simulink model "ModelEquationsDOF2"  (R2022b)
settings: Solver=ode4  StartTime=0.0  StopTime=100  FixedStep=10^-3  RelTol=1e-3
values from neighbouring files (symbols this model uses):
  cs = 900    [OptimizedParamDOF2.m]
  cu = 850    [ModelFixedParamDOF2.m]
  ks = 10039    [OptimizedParamDOF2.m]
  ku = 150000    [ModelFixedParamDOF2.m]
  ms = 237    [ModelFixedParamDOF2.m]    (also in ModelFixedParamDOF3.m = 35; ModelFixedParamDOF5.m = 730)
  mu = 20    [ModelFixedParamDOF2.m]
  road_front_wheel = M.'    [LoadRoadScript.m]
settings Model: Creator=Ade  LastModifiedBy=andre
settings SolverCC: AlgebraicLoopSolver=TrustRegion
settings DataIOCC: ReturnWorkspaceOutputs=off
settings DebuggingCC: UnconnectedInputMsg=warning  UnconnectedOutputMsg=warning  UnconnectedLineMsg=warning  SFMachineParentedDataDiag=warning  ArithmeticOperatorsInVariantConditions=warning
settings ModelReferenceCC: EnableRefExpFcnMdlSchedulingChecks=on
settings SFSimCC: SimUseLocalCustomCode=off  CustomCodeUndefinedFunction=UseInterfaceOnly
settings RTWCC: RTWUseLocalCustomCode=off  DLArmComputeVersion=19.05

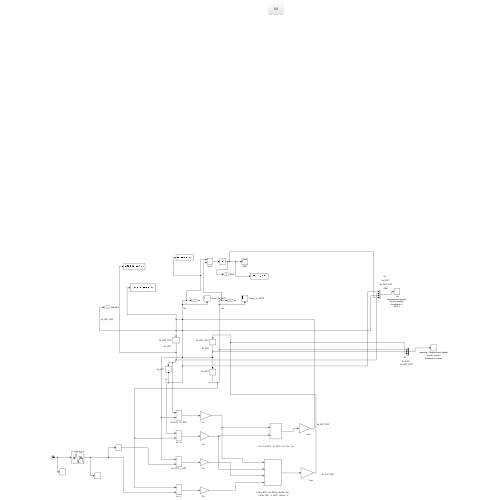
[thumbnail: Simulink's stored preview of the top-level diagram]
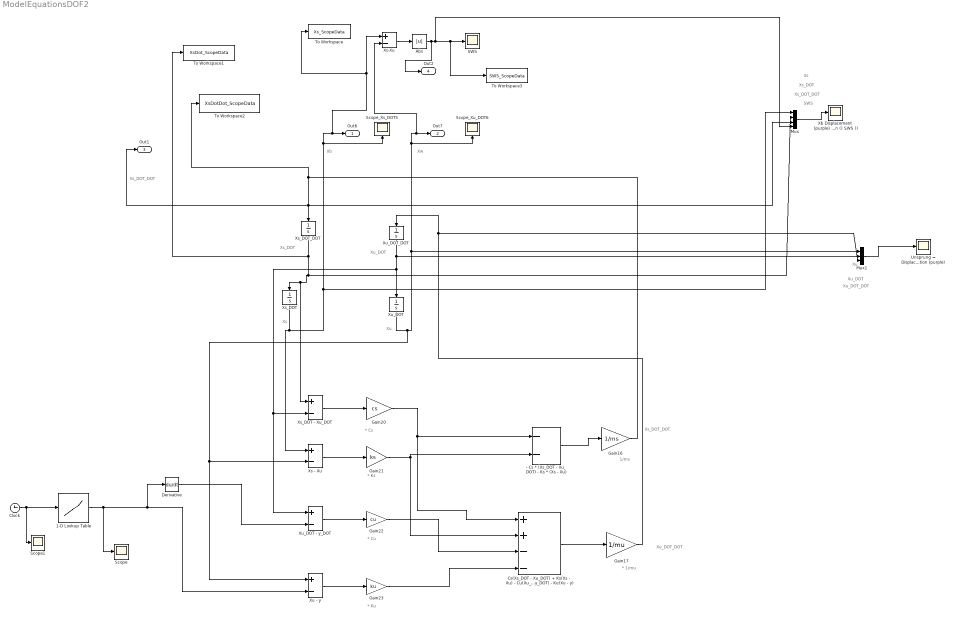
== system ModelEquationsDOF2 ==
  note: Xu_DOT_DOT
  note: * 1/mu
  note: Xs
  note: Xs_DOT
  note: Xu
  note: Xu_DOT
  note: Xu_DOT_DOT
  note: Xs_DOT_DOT
  note: 1/ms
  note: Xb
  note: Xw
  note: Xs_DOT_DOT
  note: * Ku
  note: * Cu
  note: * Cs
  note: * Ks
  note: Xu_DOT
  note: Xu
  note: Xs
  note: Xs_DOT
  note: Xs_DOT_DOT
  note: SWS
  " Cs(Xs_DOT - Xu_DOT) + Ks(Xs - Xu) - Cu(Xu_DOT - y_DOT) - Ku(Xu - y)" : Sum  Inputs=++--
  " - Cs * (Xs_DOT - Xu_DOT) - Ks * (Xs - Xu)" : Sum  Inputs=--
  "  Xb Displacement (purple) Velocity (purple) Acceleration () SWS ()" : Scope
  1-D Lookup Table : Lookup_n-D  NumberOfTableDimensions=1  LookupTableObject=road_front_wheel  BreakpointsForDimension1=[1:100]  Table=road_front_wheel  InternalRulePriority=Speed  RndMeth=Simplest
  Abs : Abs  SaturateOnIntegerOverflow=off
  Clock : Clock
  Derivative : Derivative
  Gain16 : Gain  Gain=1/ms
  Gain17 : Gain  Gain=1/mu
  Gain20 : Gain  Gain=cs
  Gain21 : Gain  Gain=ks
  Gain22 : Gain  Gain=cu
  Gain23 : Gain  Gain=ku
  Mux : Mux
  Mux1 : Mux  Inputs=3
  SWS : Scope
  Scope : Scope
  Scope1 : Scope
  Scope_Xs_DOT5 : Scope
  Scope_Xu_DOT6 : Scope
  To Workspace : ToWorkspace  VariableName=Xs_ScopeData  SaveFormat=Structure With Time  SampleTime=-1
  To Workspace1 : ToWorkspace  VariableName=XsDot_ScopeData  SaveFormat=Structure With Time  SampleTime=-1
  To Workspace2 : ToWorkspace  VariableName=XsDotDot_ScopeData  SaveFormat=Structure With Time  SampleTime=-1
  To Workspace3 : ToWorkspace  VariableName=SWS_ScopeData  SaveFormat=Structure With Time  SampleTime=-1
  Unsprung = Displacement (yellow) Velocity (purple) Acceleration (purple) : Scope
  Xs - Xu : Sum  Inputs=+-
  Xs-Xu : Sum  Inputs=+-
  Xs_DOT : Integrator
  Xs_DOT - Xu_DOT : Sum  Inputs=+-
  Xs_DOT_DOT : Integrator
  Xu - y : Sum  Inputs=+-
  "Xu_DOT " : Integrator
  "Xu_DOT - y_DOT " : Sum  Inputs=+-
  "Xu_DOT_DOT " : Integrator
  Out6 : Outport  SignalName=Xs  VectorParamsAs1DForOutWhenUnconnected=off
  Out7 : Outport  Port=2  SignalName=Xu  VectorParamsAs1DForOutWhenUnconnected=off
  Out1 : Outport  Port=3  SignalName=XsDotDot  VectorParamsAs1DForOutWhenUnconnected=off
  Out2 : Outport  Port=4  SignalName=SWS  VectorParamsAs1DForOutWhenUnconnected=off
  wires:
  Xs_DOT/1 -> Mux/1, To Workspace/1, Xs-Xu/1, Out6/1, Scope_Xs_DOT5/1, Xs - Xu/1
  " - Cs * (Xs_DOT - Xu_DOT) - Ks * (Xs - Xu)"/1 -> Gain16/1
  " Cs(Xs_DOT - Xu_DOT) + Ks(Xs - Xu) - Cu(Xu_DOT - y_DOT) - Ku(Xu - y)"/1 -> Gain17/1
  Xs - Xu/1 -> Gain21/1
  Xs_DOT - Xu_DOT/1 -> Gain20/1
  Xu - y/1 -> Gain23/1
  "Xu_DOT - y_DOT "/1 -> Gain22/1
  Gain23/1 -> " Cs(Xs_DOT - Xu_DOT) + Ks(Xs - Xu) - Cu(Xu_DOT - y_DOT) - Ku(Xu - y)"/4
  Gain22/1 -> " Cs(Xs_DOT - Xu_DOT) + Ks(Xs - Xu) - Cu(Xu_DOT - y_DOT) - Ku(Xu - y)"/3
  Gain21/1 -> " - Cs * (Xs_DOT - Xu_DOT) - Ks * (Xs - Xu)"/2, " Cs(Xs_DOT - Xu_DOT) + Ks(Xs - Xu) - Cu(Xu_DOT - y_DOT) - Ku(Xu - y)"/2
  Gain20/1 -> " - Cs * (Xs_DOT - Xu_DOT) - Ks * (Xs - Xu)"/1, " Cs(Xs_DOT - Xu_DOT) + Ks(Xs - Xu) - Cu(Xu_DOT - y_DOT) - Ku(Xu - y)"/1
  "Xu_DOT_DOT "/1 -> "Xu_DOT "/1, "Xu_DOT - y_DOT "/1, Xs_DOT - Xu_DOT/2, Mux1/2
  Gain16/1 -> Out1/1, Xs_DOT_DOT/1, Mux/3, To Workspace2/1
  Gain17/1 -> "Xu_DOT_DOT "/1, Mux1/3
  1-D Lookup Table/1 -> Scope/1, Derivative/1, Xu - y/2
  "Xu_DOT "/1 -> Mux1/1, Xs-Xu/2, Out7/1, Scope_Xu_DOT6/1, Xu - y/1, Xs - Xu/2
  Xs-Xu/1 -> Abs/1
  Mux/1 -> "  Xb Displacement (purple) Velocity (purple) Acceleration () SWS ()"/1
  Mux1/1 -> Unsprung = Displacement (yellow) Velocity (purple) Acceleration (purple)/1
  Xs_DOT_DOT/1 -> Xs_DOT - Xu_DOT/1, Xs_DOT/1, Mux/2, To Workspace1/1
  Clock/1 -> Scope1/1, 1-D Lookup Table/1
  Abs/1 -> Out2/1, Mux/4, To Workspace3/1, SWS/1
  Derivative/1 -> "Xu_DOT - y_DOT "/2
